simulink model "simulation_2014a"  (R2014a)
settings: Solver=ode45  StartTime=0.0  StopTime=1500  RelTol=1e-3
undefined symbols (not defined in the file or in its folder): model
settings Model: Creator=schauer  LastModifiedBy=schauer
settings DebuggingCC: MergeDetectMultiDrivingBlocksExec=error  FrameProcessingCompatibilityMsg=error

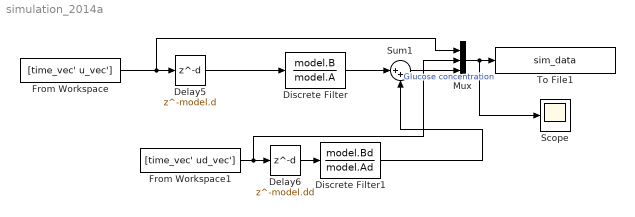
== system simulation_2014a ==
  Delay5 : Delay  DelayLength=model.d  InitialCondition=0  SampleTime=model.Ts
  Delay6 : Delay  DelayLength=model.dd  InitialCondition=0  SampleTime=model.Ts
  Discrete Filter : DiscreteFilter  Numerator=model.B  Denominator=model.A
  Discrete Filter1 : DiscreteFilter  Numerator=model.Bd  Denominator=model.Ad
  From Workspace : FromWorkspace  VariableName=[time_vec' u_vec']  SampleTime=0  Interpolate=off  OutputAfterFinalValue=Setting to zero
  From Workspace1 : FromWorkspace  VariableName=[time_vec' ud_vec']  SampleTime=0  Interpolate=off  OutputAfterFinalValue=Setting to zero
  Mux : Mux  Inputs=3
  Scope : Scope
      settings: TimeRange=auto  MaxDataPoints=5000  SaveToWorkspace=off  SaveName=ScopeData  YMin=-400.00000  YMax=600.00000  SampleTime=-1
  Sum1 : Sum  Inputs=|++
  To File1 : ToFile  Filename=sim_data  MatrixName=data  SampleTime=model.Ts
  wires:
  From Workspace1/1 -> Delay6/1, Mux/2
  From Workspace/1 -> Mux/1, Delay5/1
  Discrete Filter1/1 -> Sum1/2
  Discrete Filter/1 -> Sum1/1
  Delay6/1 -> Discrete Filter1/1
  Delay5/1 -> Discrete Filter/1
  Sum1/1 -> Mux/3  "Glucose concentration"
  Mux/1 -> Scope/1, To File1/1
